simulink model "Mass_spring_system"  (R2019a)
settings: Solver=VariableStepAuto  StartTime=0.0  StopTime=100  MaxStep=0.01  RelTol=1e-3
settings Model: Creator=91839  LastModifiedBy=shubhadam
settings DataIOCC: ExternalInput=data  LoadExternalInput=on  SaveFormat=Array  DSMLogging=off  ReturnWorkspaceOutputs=off
settings DebuggingCC: SFMachineParentedDataDiag=error

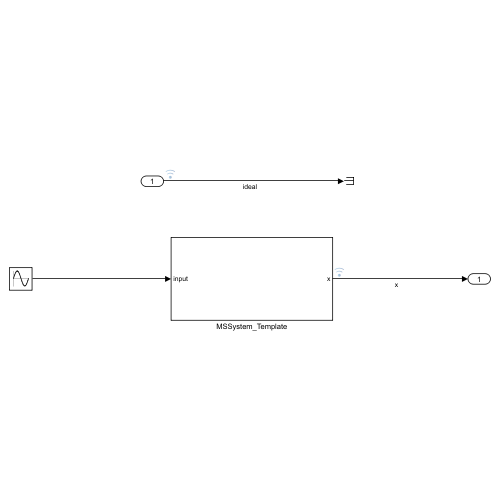
[thumbnail: Simulink's stored preview of the top-level diagram]
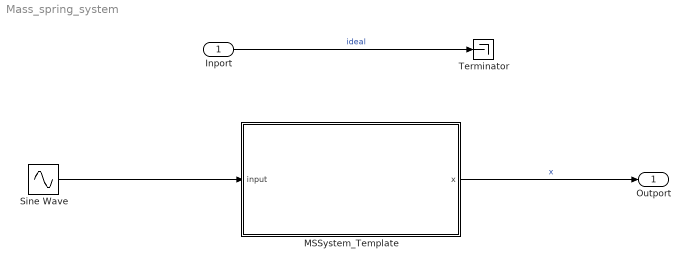
== system Mass_spring_system ==
  Inport : Inport
  MSSystem_Template : Subsystem
  Sine Wave : Sin  SampleTime=0
  Terminator : Terminator
  Outport : Outport
  wires:
  Inport/1 -> Terminator/1  "ideal"
  Sine Wave/1 -> MSSystem_Template/1(input)
  MSSystem_Template/1(x) -> Outport/1  "x"

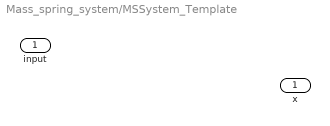
== system Mass_spring_system/MSSystem_Template ==
  input : Inport
  x : Outport
